simulink model "E6_Harmonicas"  (R2018a)
settings: Solver=VariableStepAuto  StartTime=0.0  StopTime=1  RelTol=1e-3
libraries: powerlib x17
settings Model: Creator=Rafael Pavan  LastModifiedBy=Rafael Pavan

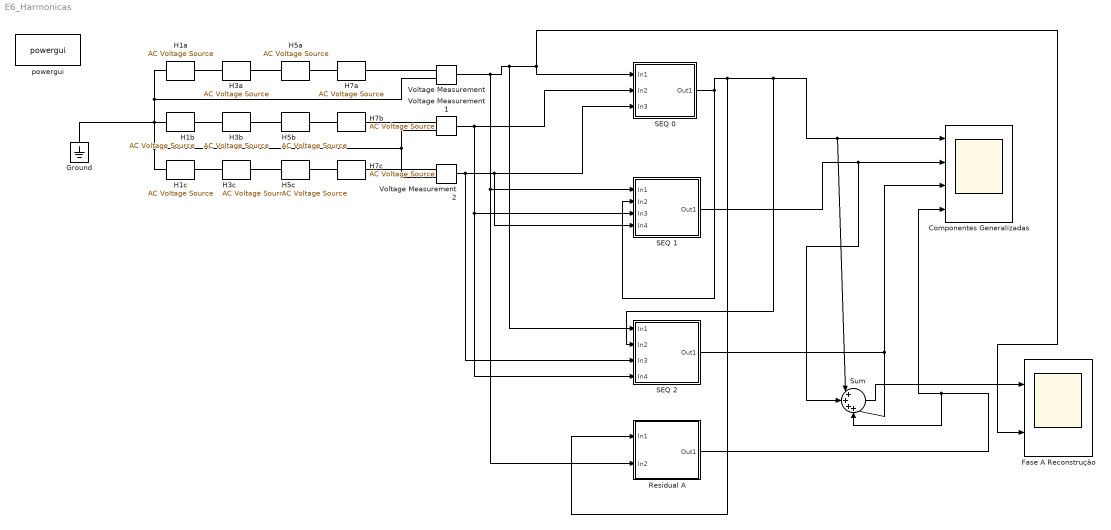
== system E6_Harmonicas ==
  Componentes Generalizadas : Scope  NumInputPorts=4
  Fase A Reconstrução : Scope  NumInputPorts=2
  Ground : powerlib/Elements/Ground  LConnTagsString=a
  H1a : powerlib/Electrical Sources/AC Voltage Source  Amplitude=100  Phase=0  Frequency=60  SampleTime=0  Measurements=None  BusType=swing  Pref=10e3  Qref=0  Qmin=-inf  Qmax=+inf
  H1b : powerlib/Electrical Sources/AC Voltage Source  Amplitude=120  Phase=-130  Frequency=60  SampleTime=0  Measurements=None  BusType=swing  Pref=10e3  Qref=0  Qmin=-inf  Qmax=+inf
  H1c : powerlib/Electrical Sources/AC Voltage Source  Amplitude=90  Phase=100  Frequency=60  SampleTime=0  Measurements=None  BusType=swing  Pref=10e3  Qref=0  Qmin=-inf  Qmax=+inf
  H3a : powerlib/Electrical Sources/AC Voltage Source  Amplitude=50  Phase=30  Frequency=180  SampleTime=0  Measurements=None  BusType=swing  Pref=10e3  Qref=0  Qmin=-inf  Qmax=+inf
  H3b : powerlib/Electrical Sources/AC Voltage Source  Amplitude=60  Phase=150  Frequency=180  SampleTime=0  Measurements=None  BusType=swing  Pref=10e3  Qref=0  Qmin=-inf  Qmax=+inf
  H3c : powerlib/Electrical Sources/AC Voltage Source  Amplitude=40  Phase=-100  Frequency=180  SampleTime=0  Measurements=None  BusType=swing  Pref=10e3  Qref=0  Qmin=-inf  Qmax=+inf
  H5a : powerlib/Electrical Sources/AC Voltage Source  Amplitude=30  Phase=0  Frequency=300  SampleTime=0  Measurements=None  BusType=swing  Pref=10e3  Qref=0  Qmin=-inf  Qmax=+inf
  H5b : powerlib/Electrical Sources/AC Voltage Source  Amplitude=20  Phase=125  Frequency=300  SampleTime=0  Measurements=None  BusType=swing  Pref=10e3  Qref=0  Qmin=-inf  Qmax=+inf
  H5c : powerlib/Electrical Sources/AC Voltage Source  Amplitude=10  Phase=-90  Frequency=300  SampleTime=0  Measurements=None  BusType=swing  Pref=10e3  Qref=0  Qmin=-inf  Qmax=+inf
  H7a : powerlib/Electrical Sources/AC Voltage Source  Amplitude=15  Phase=20  Frequency=420  SampleTime=0  Measurements=None  BusType=swing  Pref=10e3  Qref=0  Qmin=-inf  Qmax=+inf
  H7b : powerlib/Electrical Sources/AC Voltage Source  Amplitude=8  Phase=-150  Frequency=420  SampleTime=0  Measurements=None  BusType=swing  Pref=10e3  Qref=0  Qmin=-inf  Qmax=+inf
  H7c : powerlib/Electrical Sources/AC Voltage Source  Amplitude=10  Phase=200  Frequency=420  SampleTime=0  Measurements=None  BusType=swing  Pref=10e3  Qref=0  Qmin=-inf  Qmax=+inf
  Residual A : Subsystem
  SEQ 0 : Subsystem
  SEQ 1 : Subsystem
  "SEQ 2 " : Subsystem
  Sum : Sum  Inputs=|++++
  Voltage Measurement : powerlib/Measurements/Voltage Measurement  PhasorSimulation=off  OutputType=Complex  PSBequivalent=0
  Voltage Measurement1 : powerlib/Measurements/Voltage Measurement  PhasorSimulation=off  OutputType=Complex  PSBequivalent=0
  Voltage Measurement2 : powerlib/Measurements/Voltage Measurement  PhasorSimulation=off  OutputType=Complex  PSBequivalent=0
  powergui : powerlib/powergui  Priority=1  SimulationMode=Continuous  SampleTime=50e-6  frequency=60  Iterations=50  frequencyindice=60  Pbase=100e6  ErrMax=1e-4  UnitsV=kV  UnitsW=MW  buscounter=0  FunctionMessages=off  echomessages=off  EnableUseOfTLC=off  CurrentSourceSwitches=off  DisableSnubberDevices=off  DisableRonSwitches=off  DisableVfSwitches=off  DisplayEquations=off  SolverType=Tustin/Backward Euler (TBE)  Interpol=off  ExternalGateDelay=off  methode=off  Ts=100  x0status=blocks  SPID=on  SwTol=0  HookPort=off  RestoreLinks=warning  ResistiveCurrentMeasurement=off  Frange=[0:2:500]  Ylog=off  Xlog=on  ShowGrid=off  save=off  variable=ZData  structure=GZS1  ZoomFFT=off  StartTime=0.5  cycles=20  DisplayStyle=2  fundamental=60  FreqAxis=off  MaxFrequency=1000  frequencyindicesteady=1  RmsSteady=1  display=off
  wires:
  Sum/1 -> Fase A Reconstrução/1
  Voltage Measurement/1 -> Residual A/2(In2), SEQ 1/1(In1), "SEQ 2 "/1(In1), Fase A Reconstrução/2, SEQ 0/1(In1)
  Voltage Measurement1/1 -> "SEQ 2 "/4(In4), SEQ 1/3(In3), SEQ 0/2(In2)
  Voltage Measurement2/1 -> "SEQ 2 "/3(In3), SEQ 1/4(In4), SEQ 0/3(In3)
  SEQ 0/1(Out1) -> Residual A/1(In1), "SEQ 2 "/2(In2), Componentes Generalizadas/1, Sum/1, SEQ 1/2(In2)
  SEQ 1/1(Out1) -> Sum/2, Componentes Generalizadas/2
  "SEQ 2 "/1(Out1) -> Componentes Generalizadas/3, Sum/3
  Residual A/1(Out1) -> Componentes Generalizadas/4, Sum/4
  connections:
  H3a/LConn1 -- H1a/RConn1
  H5a/LConn1 -- H3a/RConn1
  H7a/LConn1 -- H5a/RConn1
  H7b/LConn1 -- H5b/RConn1
  H3b/LConn1 -- H1b/RConn1
  H5b/LConn1 -- H3b/RConn1
  H7c/LConn1 -- H5c/RConn1
  H3c/LConn1 -- H1c/RConn1
  H5c/LConn1 -- H3c/RConn1
  H7a/RConn1 -- Voltage Measurement/LConn1
  H1a/LConn1 -- Voltage Measurement/LConn2 -- Ground/LConn1 -- Voltage Measurement1/LConn2 -- Voltage Measurement2/LConn2 -- H1c/LConn1 -- H1b/LConn1
  Voltage Measurement1/LConn1 -- H7b/RConn1
  Voltage Measurement2/LConn1 -- H7c/RConn1

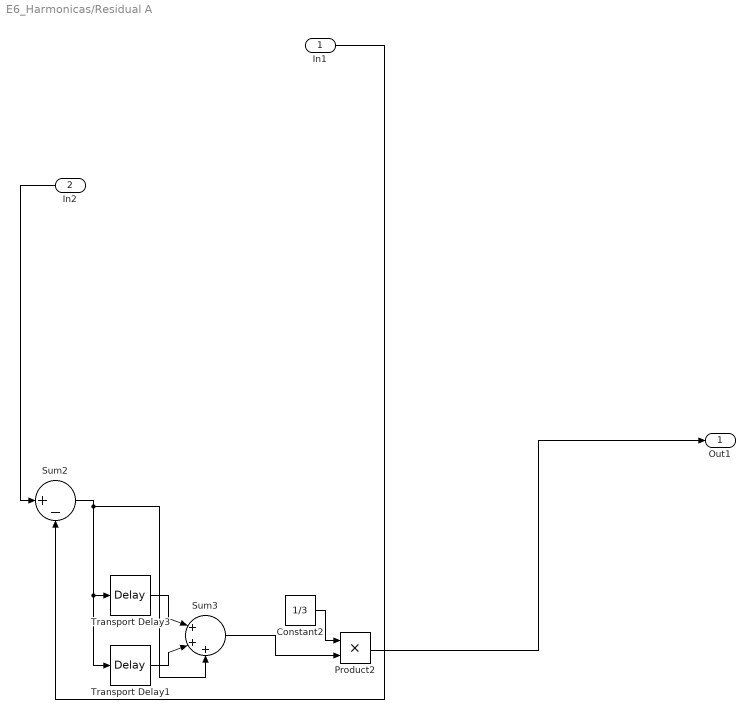
== system E6_Harmonicas/Residual A ==
  In1 : Inport
  In2 : Inport  Port=2
  Constant2 : Constant  Value=1/3
  Product2 : Product
  Sum2 : Sum  Inputs=|+-
  Sum3 : Sum  Inputs=|+++
  Transport Delay1 : TransportDelay  DelayTime=(1/60)/3
  Transport Delay3 : TransportDelay  DelayTime=2*(1/60)/3
  Out1 : Outport
  wires:
  Transport Delay1/1 -> Sum3/2
  Transport Delay3/1 -> Sum3/1
  Constant2/1 -> Product2/1
  Sum2/1 -> Sum3/3, Transport Delay1/1, Transport Delay3/1
  In1/1 -> Sum2/2
  Sum3/1 -> Product2/2
  Product2/1 -> Out1/1
  In2/1 -> Sum2/1

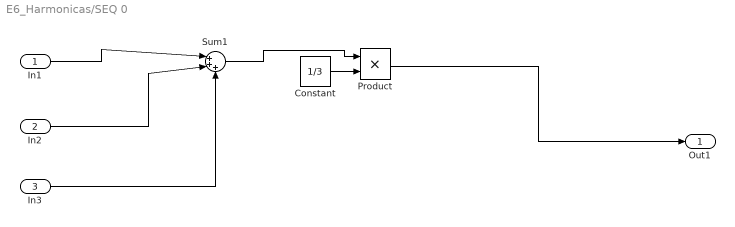
== system E6_Harmonicas/SEQ 0 ==
  In1 : Inport
  In2 : Inport  Port=2
  In3 : Inport  Port=3
  Constant : Constant  Value=1/3
  Product : Product
  Sum1 : Sum  Inputs=|+++
  Out1 : Outport
  wires:
  Constant/1 -> Product/2
  In3/1 -> Sum1/3
  Sum1/1 -> Product/1
  Product/1 -> Out1/1
  In2/1 -> Sum1/2
  In1/1 -> Sum1/1

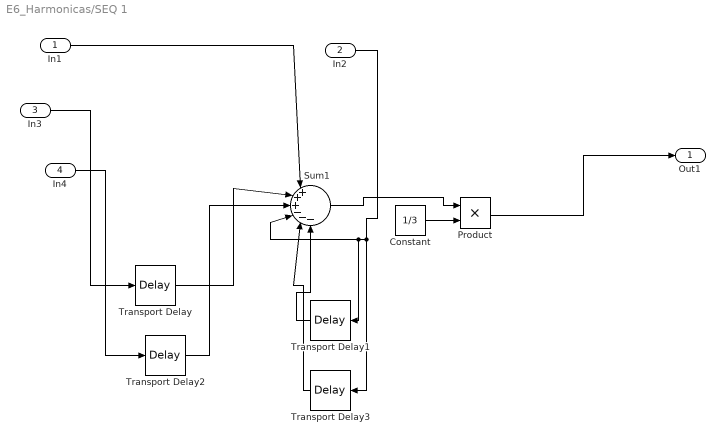
== system E6_Harmonicas/SEQ 1 ==
  In1 : Inport
  In2 : Inport  Port=2
  In3 : Inport  Port=3
  In4 : Inport  Port=4
  Constant : Constant  Value=1/3
  Product : Product
  Sum1 : Sum  Inputs=|+++---
  Transport Delay : TransportDelay  DelayTime=(1/60)/3
  Transport Delay1 : TransportDelay  DelayTime=(1/60)/3
  Transport Delay2 : TransportDelay  DelayTime=2*(1/60)/3
  Transport Delay3 : TransportDelay  DelayTime=2*(1/60)/3
  Out1 : Outport
  wires:
  Transport Delay2/1 -> Sum1/3
  Product/1 -> Out1/1
  In2/1 -> Transport Delay3/1, Transport Delay1/1, Sum1/4
  Constant/1 -> Product/2
  Transport Delay3/1 -> Sum1/5
  Sum1/1 -> Product/1
  Transport Delay/1 -> Sum1/2
  In3/1 -> Transport Delay/1
  Transport Delay1/1 -> Sum1/6
  In4/1 -> Transport Delay2/1
  In1/1 -> Sum1/1

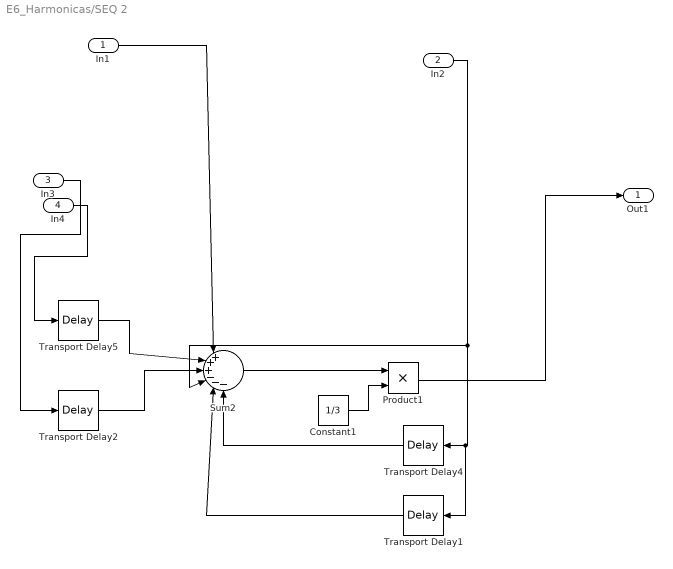
== system E6_Harmonicas/SEQ 2  ==
  In1 : Inport
  In2 : Inport  Port=2
  In3 : Inport  Port=3
  In4 : Inport  Port=4
  Constant1 : Constant  Value=1/3
  Product1 : Product
  Sum2 : Sum  Inputs=|+++---
  Transport Delay1 : TransportDelay  DelayTime=(1/60)/3
  Transport Delay2 : TransportDelay  DelayTime=(1/60)/3
  Transport Delay4 : TransportDelay  DelayTime=2*(1/60)/3
  Transport Delay5 : TransportDelay  DelayTime=2*(1/60)/3
  Out1 : Outport
  wires:
  Transport Delay1/1 -> Sum2/5
  In2/1 -> Sum2/4, Transport Delay1/1, Transport Delay4/1
  In1/1 -> Sum2/1
  Transport Delay4/1 -> Sum2/6
  Transport Delay2/1 -> Sum2/3
  Sum2/1 -> Product1/1
  In3/1 -> Transport Delay2/1
  Constant1/1 -> Product1/2
  Transport Delay5/1 -> Sum2/2
  Product1/1 -> Out1/1
  In4/1 -> Transport Delay5/1
